simulink model "BLOCK_SEVEN_TAP_FILTER"  (R2022b)
settings: Solver=FixedStepDiscrete  StartTime=0.0  StopTime=10.0  RelTol=1e-3
libraries: dspsrcs4 x1
settings Model: DataTypeOverride=Off  Creator=saran  LastModifiedBy=saran
settings SolverCC: AlgebraicLoopSolver=TrustRegion
settings DataIOCC: LimitDataPoints=on  SaveOutput=off  SaveTime=off
settings OptimizationCC: BlockReduction=off  ConditionallyExecuteInputs=off  DefaultParameterBehavior=Inlined  DefaultUnderspecifiedDataType=single  LifeSpan=inf
settings DebuggingCC: AlgebraicLoopMsg=error  SingleTaskRateTransMsg=error  UnconnectedInputMsg=warning  UnconnectedOutputMsg=warning  UnconnectedLineMsg=warning  AllowSymbolicDim=off  StrictBusMsg=ErrorOnBusTreatedAsVector  SFUnexpectedBacktrackingDiag=warning  SFNoUnconditionalDefaultTransitionDiag=warning  SFExecutionAtInitializationDiag=none  SFMachineParentedDataDiag=warning  ArithmeticOperatorsInVariantConditions=warning
settings HardwareCC: ProdBitPerPointer=32  ProdBitPerSizeT=32  ProdBitPerPtrDiffT=32  ProdLargestAtomicFloat=None  ProdIntDivRoundTo=Undefined  ProdEndianess=Unspecified  ProdWordSize=32  ProdHWDeviceType=ASIC/FPGA->ASIC/FPGA  ProdEqTarget=off
settings ModelReferenceCC: EnableRefExpFcnMdlSchedulingChecks=on
settings SFSimCC: SimUseLocalCustomCode=off  CustomCodeUndefinedFunction=UseInterfaceOnly
settings RTWCC: RTWUseLocalCustomCode=off
settings CodeAppCC: StateflowObjectComments=on
settings GRTTargetCC: TargetLangStandard=C89/C90 (ANSI)
settings ConfigComp: CovScope=ReferencedModels  CovMetricSettings=dw  CovSaveCumulativeToWorkspaceVar=on  CovSaveSingleToWorkspaceVar=on  CovExternalEMLEnable=off  CovSFcnEnable=off

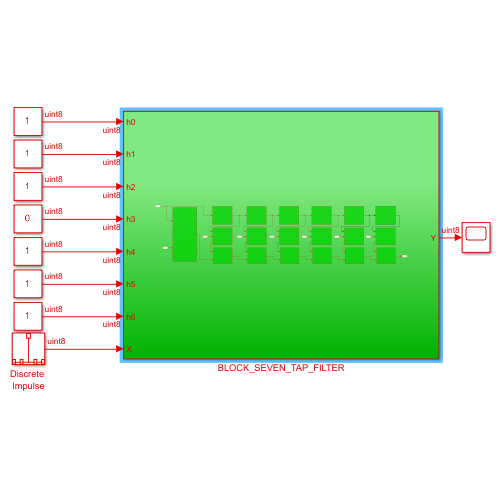
[thumbnail: Simulink's stored preview of the top-level diagram]
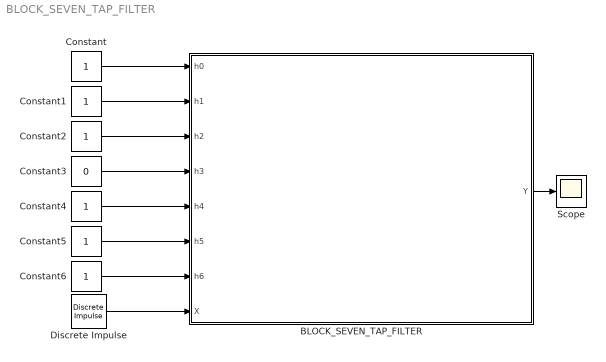
== system BLOCK_SEVEN_TAP_FILTER ==
  BLOCK_SEVEN_TAP_FILTER : Subsystem
  Constant{,1..2,4..6} (6 alike) : Constant  OutDataTypeStr=uint8  SampleTime=1
  Constant3 : Constant  Value=0  OutDataTypeStr=uint8  SampleTime=1
  Discrete Impulse : dspsrcs4/Discrete  Impulse  Delay=0  SampleTime=1  FrameSample=1  OutputFrames=off  dataType=uint8  isSigned=on  wordLen=16  udDataType=sfix(16)  fracBitsMode=Best precision  numFracBits=15  OutDataTypeStr=uint8  LastOutDataTypeStr=uint8
  Scope : Scope
  wires:
  Constant6/1 -> BLOCK_SEVEN_TAP_FILTER/7(h6)
  Constant/1 -> BLOCK_SEVEN_TAP_FILTER/1(h0)
  Constant1/1 -> BLOCK_SEVEN_TAP_FILTER/2(h1)
  Constant2/1 -> BLOCK_SEVEN_TAP_FILTER/3(h2)
  Constant3/1 -> BLOCK_SEVEN_TAP_FILTER/4(h3)
  Constant4/1 -> BLOCK_SEVEN_TAP_FILTER/5(h4)
  Constant5/1 -> BLOCK_SEVEN_TAP_FILTER/6(h5)
  Discrete Impulse/1 -> BLOCK_SEVEN_TAP_FILTER/8(X)
  BLOCK_SEVEN_TAP_FILTER/1(Y) -> Scope/1

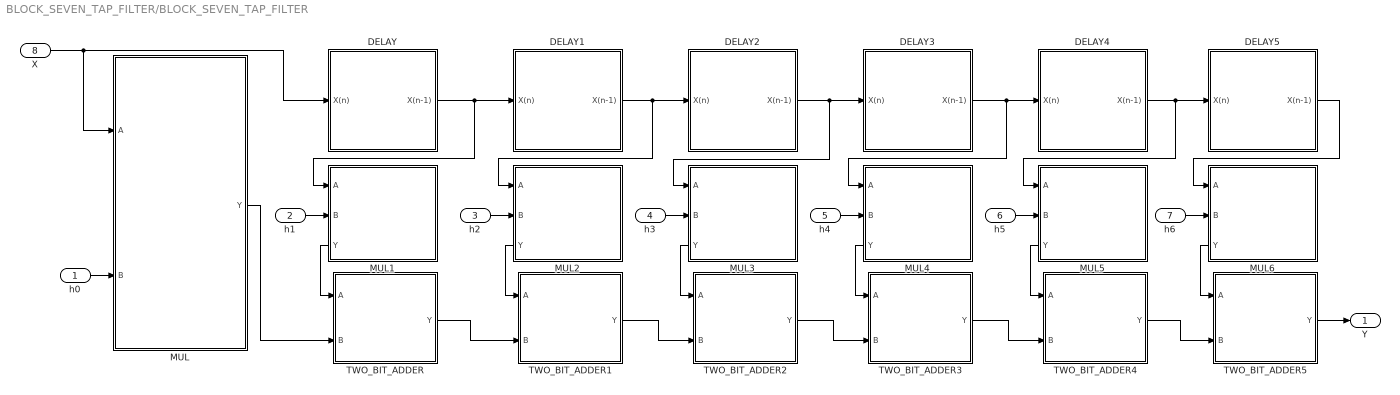
== system BLOCK_SEVEN_TAP_FILTER/BLOCK_SEVEN_TAP_FILTER ==
  h0 : Inport  OutDataTypeStr=uint8  SampleTime=1
  h1 : Inport  Port=2  OutDataTypeStr=uint8  SampleTime=1
  h2 : Inport  Port=3  OutDataTypeStr=uint8  SampleTime=1
  h3 : Inport  Port=4  OutDataTypeStr=uint8  SampleTime=1
  h4 : Inport  Port=5  OutDataTypeStr=uint8  SampleTime=1
  h5 : Inport  Port=6  OutDataTypeStr=uint8  SampleTime=1
  h6 : Inport  Port=7  OutDataTypeStr=uint8  SampleTime=1
  X : Inport  Port=8
  DELAY : Subsystem
  DELAY1 : Subsystem
  DELAY2 : Subsystem
  DELAY3 : Subsystem
  DELAY4 : Subsystem
  DELAY5 : Subsystem
  MUL : Subsystem
  MUL1 : Subsystem
      settings: PortSchema="{\"entries\":[{\"content\":{\"sides\":[{\"content\":{\"connectorIds\":[\"In1\",\"In2\",\"Out1\"]},\"type\":\"ConnectorPlacement.EquallySpacedRectSide\",\"uuid\":\"6d4885f8-73c5-433a-aace-af648e409d6b\"},{\"content\":{\"connectorIds\":[],\"side\":\"RIGHT\"},\"type\":\"ConnectorPlacement.EquallySpacedRectSide\",\"uuid\":\"836fe19b-05d9-46e4-8d72-fd0891ed8906\"},{\"content\":{\"connectorIds\":[],\"side\":\"TOP\"},\"type\":\"ConnectorPlacement.EquallySpacedRectSide\",\"uuid\":\"c1eb711e-365c-41f2-92fe-7283fb1d6e9c\"}]},\"type\":\"ConnectorPlacement.EquallySpacedConnector\",\"uuid\":\"b7c1d480-b729-42dd-8c7b-e0a62792d202\"}],\"packageUris\":[\"http://schema.mathworks.com/mf0/Connector/R2020b\"],\"version\":\"1.0\"}"
  MUL2 : Subsystem
      settings: PortSchema="{\"entries\":[{\"content\":{\"sides\":[{\"content\":{\"connectorIds\":[\"In1\",\"In2\",\"Out1\"]},\"type\":\"ConnectorPlacement.EquallySpacedRectSide\",\"uuid\":\"6d4885f8-73c5-433a-aace-af648e409d6b\"},{\"content\":{\"connectorIds\":[],\"side\":\"RIGHT\"},\"type\":\"ConnectorPlacement.EquallySpacedRectSide\",\"uuid\":\"836fe19b-05d9-46e4-8d72-fd0891ed8906\"},{\"content\":{\"connectorIds\":[],\"side\":\"TOP\"},\"type\":\"ConnectorPlacement.EquallySpacedRectSide\",\"uuid\":\"c1eb711e-365c-41f2-92fe-7283fb1d6e9c\"}]},\"type\":\"ConnectorPlacement.EquallySpacedConnector\",\"uuid\":\"b7c1d480-b729-42dd-8c7b-e0a62792d202\"}],\"packageUris\":[\"http://schema.mathworks.com/mf0/Connector/R2020b\"],\"version\":\"1.0\"}"
  MUL3 : Subsystem
      settings: PortSchema="{\"entries\":[{\"content\":{\"sides\":[{\"content\":{\"connectorIds\":[\"In1\",\"In2\",\"Out1\"]},\"type\":\"ConnectorPlacement.EquallySpacedRectSide\",\"uuid\":\"6d4885f8-73c5-433a-aace-af648e409d6b\"},{\"content\":{\"connectorIds\":[],\"side\":\"RIGHT\"},\"type\":\"ConnectorPlacement.EquallySpacedRectSide\",\"uuid\":\"836fe19b-05d9-46e4-8d72-fd0891ed8906\"},{\"content\":{\"connectorIds\":[],\"side\":\"TOP\"},\"type\":\"ConnectorPlacement.EquallySpacedRectSide\",\"uuid\":\"c1eb711e-365c-41f2-92fe-7283fb1d6e9c\"}]},\"type\":\"ConnectorPlacement.EquallySpacedConnector\",\"uuid\":\"b7c1d480-b729-42dd-8c7b-e0a62792d202\"}],\"packageUris\":[\"http://schema.mathworks.com/mf0/Connector/R2020b\"],\"version\":\"1.0\"}"
  MUL4 : Subsystem
      settings: PortSchema="{\"entries\":[{\"content\":{\"sides\":[{\"content\":{\"connectorIds\":[\"In1\",\"In2\",\"Out1\"]},\"type\":\"ConnectorPlacement.EquallySpacedRectSide\",\"uuid\":\"6d4885f8-73c5-433a-aace-af648e409d6b\"},{\"content\":{\"connectorIds\":[],\"side\":\"RIGHT\"},\"type\":\"ConnectorPlacement.EquallySpacedRectSide\",\"uuid\":\"836fe19b-05d9-46e4-8d72-fd0891ed8906\"},{\"content\":{\"connectorIds\":[],\"side\":\"TOP\"},\"type\":\"ConnectorPlacement.EquallySpacedRectSide\",\"uuid\":\"c1eb711e-365c-41f2-92fe-7283fb1d6e9c\"}]},\"type\":\"ConnectorPlacement.EquallySpacedConnector\",\"uuid\":\"b7c1d480-b729-42dd-8c7b-e0a62792d202\"}],\"packageUris\":[\"http://schema.mathworks.com/mf0/Connector/R2020b\"],\"version\":\"1.0\"}"
  MUL5 : Subsystem
      settings: PortSchema="{\"entries\":[{\"content\":{\"sides\":[{\"content\":{\"connectorIds\":[\"In1\",\"In2\",\"Out1\"]},\"type\":\"ConnectorPlacement.EquallySpacedRectSide\",\"uuid\":\"6d4885f8-73c5-433a-aace-af648e409d6b\"},{\"content\":{\"connectorIds\":[],\"side\":\"RIGHT\"},\"type\":\"ConnectorPlacement.EquallySpacedRectSide\",\"uuid\":\"836fe19b-05d9-46e4-8d72-fd0891ed8906\"},{\"content\":{\"connectorIds\":[],\"side\":\"TOP\"},\"type\":\"ConnectorPlacement.EquallySpacedRectSide\",\"uuid\":\"c1eb711e-365c-41f2-92fe-7283fb1d6e9c\"}]},\"type\":\"ConnectorPlacement.EquallySpacedConnector\",\"uuid\":\"b7c1d480-b729-42dd-8c7b-e0a62792d202\"}],\"packageUris\":[\"http://schema.mathworks.com/mf0/Connector/R2020b\"],\"version\":\"1.0\"}"
  MUL6 : Subsystem
      settings: PortSchema="{\"entries\":[{\"content\":{\"sides\":[{\"content\":{\"connectorIds\":[\"In1\",\"In2\",\"Out1\"]},\"type\":\"ConnectorPlacement.EquallySpacedRectSide\",\"uuid\":\"6d4885f8-73c5-433a-aace-af648e409d6b\"},{\"content\":{\"connectorIds\":[],\"side\":\"RIGHT\"},\"type\":\"ConnectorPlacement.EquallySpacedRectSide\",\"uuid\":\"836fe19b-05d9-46e4-8d72-fd0891ed8906\"},{\"content\":{\"connectorIds\":[],\"side\":\"TOP\"},\"type\":\"ConnectorPlacement.EquallySpacedRectSide\",\"uuid\":\"c1eb711e-365c-41f2-92fe-7283fb1d6e9c\"}]},\"type\":\"ConnectorPlacement.EquallySpacedConnector\",\"uuid\":\"b7c1d480-b729-42dd-8c7b-e0a62792d202\"}],\"packageUris\":[\"http://schema.mathworks.com/mf0/Connector/R2020b\"],\"version\":\"1.0\"}"
  TWO_BIT_ADDER : Subsystem
  TWO_BIT_ADDER1 : Subsystem
  TWO_BIT_ADDER2 : Subsystem
  TWO_BIT_ADDER3 : Subsystem
  TWO_BIT_ADDER4 : Subsystem
  TWO_BIT_ADDER5 : Subsystem
  Y : Outport  VectorParamsAs1DForOutWhenUnconnected=off
  wires:
  h1/1 -> MUL1/2(B)
  MUL1/1(Y) -> TWO_BIT_ADDER/1(A)
  MUL2/1(Y) -> TWO_BIT_ADDER1/1(A)
  h2/1 -> MUL2/2(B)
  MUL3/1(Y) -> TWO_BIT_ADDER2/1(A)
  h3/1 -> MUL3/2(B)
  MUL4/1(Y) -> TWO_BIT_ADDER3/1(A)
  h4/1 -> MUL4/2(B)
  MUL5/1(Y) -> TWO_BIT_ADDER4/1(A)
  h5/1 -> MUL5/2(B)
  MUL6/1(Y) -> TWO_BIT_ADDER5/1(A)
  h6/1 -> MUL6/2(B)
  MUL/1(Y) -> TWO_BIT_ADDER/2(B)
  DELAY/1(X(n-1)) -> MUL1/1(A), DELAY1/1(X(n))
  TWO_BIT_ADDER/1(Y) -> TWO_BIT_ADDER1/2(B)
  DELAY1/1(X(n-1)) -> DELAY2/1(X(n)), MUL2/1(A)
  DELAY2/1(X(n-1)) -> MUL3/1(A), DELAY3/1(X(n))
  DELAY3/1(X(n-1)) -> MUL4/1(A), DELAY4/1(X(n))
  TWO_BIT_ADDER1/1(Y) -> TWO_BIT_ADDER2/2(B)
  TWO_BIT_ADDER2/1(Y) -> TWO_BIT_ADDER3/2(B)
  TWO_BIT_ADDER3/1(Y) -> TWO_BIT_ADDER4/2(B)
  TWO_BIT_ADDER4/1(Y) -> TWO_BIT_ADDER5/2(B)
  X/1 -> DELAY/1(X(n)), MUL/1(A)
  h0/1 -> MUL/2(B)
  TWO_BIT_ADDER5/1(Y) -> Y/1
  DELAY4/1(X(n-1)) -> MUL5/1(A), DELAY5/1(X(n))
  DELAY5/1(X(n-1)) -> MUL6/1(A)

== system BLOCK_SEVEN_TAP_FILTER/BLOCK_SEVEN_TAP_FILTER/DELAY ==
  X(n) : Inport  OutDataTypeStr=uint8  SampleTime=1  LockScale=on
  Delay : Delay  DelayLength=1  InitialCondition=0
  X(n-1) : Outport  OutDataTypeStr=uint8  SampleTime=1  VectorParamsAs1DForOutWhenUnconnected=off  LockScale=on
  wires:
  X(n)/1 -> Delay/1
  Delay/1 -> X(n-1)/1

== system BLOCK_SEVEN_TAP_FILTER/BLOCK_SEVEN_TAP_FILTER/DELAY1 ==
  X(n) : Inport  OutDataTypeStr=uint8  SampleTime=1  LockScale=on
  Delay : Delay  DelayLength=1  InitialCondition=0
  X(n-1) : Outport  OutDataTypeStr=uint8  SampleTime=1  VectorParamsAs1DForOutWhenUnconnected=off  LockScale=on
  wires:
  X(n)/1 -> Delay/1
  Delay/1 -> X(n-1)/1

== system BLOCK_SEVEN_TAP_FILTER/BLOCK_SEVEN_TAP_FILTER/DELAY2 ==
  X(n) : Inport  OutDataTypeStr=uint8  SampleTime=1  LockScale=on
  Delay : Delay  DelayLength=1  InitialCondition=0
  X(n-1) : Outport  OutDataTypeStr=uint8  SampleTime=1  VectorParamsAs1DForOutWhenUnconnected=off  LockScale=on
  wires:
  X(n)/1 -> Delay/1
  Delay/1 -> X(n-1)/1

== system BLOCK_SEVEN_TAP_FILTER/BLOCK_SEVEN_TAP_FILTER/DELAY3 ==
  X(n) : Inport  OutDataTypeStr=uint8  SampleTime=1  LockScale=on
  Delay : Delay  DelayLength=1  InitialCondition=0
  X(n-1) : Outport  OutDataTypeStr=uint8  SampleTime=1  VectorParamsAs1DForOutWhenUnconnected=off  LockScale=on
  wires:
  X(n)/1 -> Delay/1
  Delay/1 -> X(n-1)/1

== system BLOCK_SEVEN_TAP_FILTER/BLOCK_SEVEN_TAP_FILTER/DELAY4 ==
  X(n) : Inport  OutDataTypeStr=uint8  SampleTime=1  LockScale=on
  Delay : Delay  DelayLength=1  InitialCondition=0
  X(n-1) : Outport  OutDataTypeStr=uint8  SampleTime=1  VectorParamsAs1DForOutWhenUnconnected=off  LockScale=on
  wires:
  X(n)/1 -> Delay/1
  Delay/1 -> X(n-1)/1

== system BLOCK_SEVEN_TAP_FILTER/BLOCK_SEVEN_TAP_FILTER/DELAY5 ==
  X(n) : Inport  OutDataTypeStr=uint8  SampleTime=1  LockScale=on
  Delay : Delay  DelayLength=1  InitialCondition=0
  X(n-1) : Outport  OutDataTypeStr=uint8  SampleTime=1  VectorParamsAs1DForOutWhenUnconnected=off  LockScale=on
  wires:
  X(n)/1 -> Delay/1
  Delay/1 -> X(n-1)/1

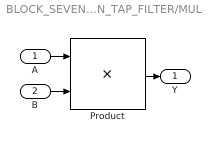
== system BLOCK_SEVEN_TAP_FILTER/BLOCK_SEVEN_TAP_FILTER/MUL ==
  A : Inport  OutDataTypeStr=uint8  SampleTime=1
  B : Inport  Port=2  OutDataTypeStr=uint8  SampleTime=1
  Product : Product  OutDataTypeStr=uint8  LockScale=on
  Y : Outport  OutDataTypeStr=uint8  SampleTime=1  VectorParamsAs1DForOutWhenUnconnected=off
  wires:
  A/1 -> Product/1
  Product/1 -> Y/1
  B/1 -> Product/2

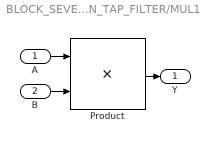
== system BLOCK_SEVEN_TAP_FILTER/BLOCK_SEVEN_TAP_FILTER/MUL1 ==
  A : Inport  OutDataTypeStr=uint8  SampleTime=1
  B : Inport  Port=2  OutDataTypeStr=uint8  SampleTime=1
  Product : Product  OutDataTypeStr=uint8  LockScale=on
  Y : Outport  OutDataTypeStr=uint8  SampleTime=1  VectorParamsAs1DForOutWhenUnconnected=off
  wires:
  A/1 -> Product/1
  Product/1 -> Y/1
  B/1 -> Product/2

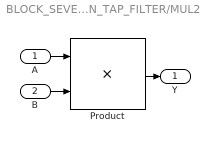
== system BLOCK_SEVEN_TAP_FILTER/BLOCK_SEVEN_TAP_FILTER/MUL2 ==
  A : Inport  OutDataTypeStr=uint8  SampleTime=1
  B : Inport  Port=2  OutDataTypeStr=uint8  SampleTime=1
  Product : Product  OutDataTypeStr=uint8  LockScale=on
  Y : Outport  OutDataTypeStr=uint8  SampleTime=1  VectorParamsAs1DForOutWhenUnconnected=off
  wires:
  A/1 -> Product/1
  Product/1 -> Y/1
  B/1 -> Product/2

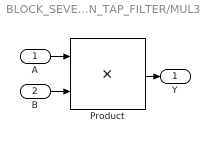
== system BLOCK_SEVEN_TAP_FILTER/BLOCK_SEVEN_TAP_FILTER/MUL3 ==
  A : Inport  OutDataTypeStr=uint8  SampleTime=1
  B : Inport  Port=2  OutDataTypeStr=uint8  SampleTime=1
  Product : Product  OutDataTypeStr=uint8  LockScale=on
  Y : Outport  OutDataTypeStr=uint8  SampleTime=1  VectorParamsAs1DForOutWhenUnconnected=off
  wires:
  A/1 -> Product/1
  Product/1 -> Y/1
  B/1 -> Product/2

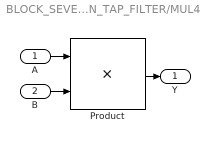
== system BLOCK_SEVEN_TAP_FILTER/BLOCK_SEVEN_TAP_FILTER/MUL4 ==
  A : Inport  OutDataTypeStr=uint8  SampleTime=1
  B : Inport  Port=2  OutDataTypeStr=uint8  SampleTime=1
  Product : Product  OutDataTypeStr=uint8  LockScale=on
  Y : Outport  OutDataTypeStr=uint8  SampleTime=1  VectorParamsAs1DForOutWhenUnconnected=off
  wires:
  A/1 -> Product/1
  Product/1 -> Y/1
  B/1 -> Product/2

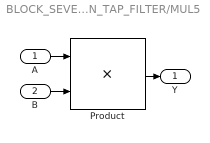
== system BLOCK_SEVEN_TAP_FILTER/BLOCK_SEVEN_TAP_FILTER/MUL5 ==
  A : Inport  OutDataTypeStr=uint8  SampleTime=1
  B : Inport  Port=2  OutDataTypeStr=uint8  SampleTime=1
  Product : Product  OutDataTypeStr=uint8  LockScale=on
  Y : Outport  OutDataTypeStr=uint8  SampleTime=1  VectorParamsAs1DForOutWhenUnconnected=off
  wires:
  A/1 -> Product/1
  Product/1 -> Y/1
  B/1 -> Product/2

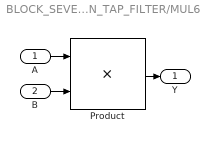
== system BLOCK_SEVEN_TAP_FILTER/BLOCK_SEVEN_TAP_FILTER/MUL6 ==
  A : Inport  OutDataTypeStr=uint8  SampleTime=1
  B : Inport  Port=2  OutDataTypeStr=uint8  SampleTime=1
  Product : Product  OutDataTypeStr=uint8  LockScale=on
  Y : Outport  OutDataTypeStr=uint8  SampleTime=1  VectorParamsAs1DForOutWhenUnconnected=off
  wires:
  A/1 -> Product/1
  Product/1 -> Y/1
  B/1 -> Product/2

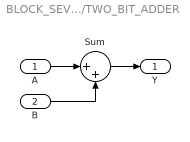
== system BLOCK_SEVEN_TAP_FILTER/BLOCK_SEVEN_TAP_FILTER/TWO_BIT_ADDER ==
  A : Inport  OutDataTypeStr=uint8
  B : Inport  Port=2  OutDataTypeStr=uint8  SampleTime=1
  Sum : Sum  Inputs=|++  OutDataTypeStr=uint8  LockScale=on
  Y : Outport  OutDataTypeStr=uint8  SampleTime=1  VectorParamsAs1DForOutWhenUnconnected=off
  wires:
  Sum/1 -> Y/1
  A/1 -> Sum/1
  B/1 -> Sum/2

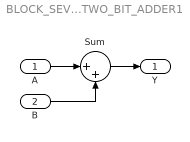
== system BLOCK_SEVEN_TAP_FILTER/BLOCK_SEVEN_TAP_FILTER/TWO_BIT_ADDER1 ==
  A : Inport  OutDataTypeStr=uint8
  B : Inport  Port=2  OutDataTypeStr=uint8  SampleTime=1
  Sum : Sum  Inputs=|++  OutDataTypeStr=uint8  LockScale=on
  Y : Outport  OutDataTypeStr=uint8  SampleTime=1  VectorParamsAs1DForOutWhenUnconnected=off
  wires:
  Sum/1 -> Y/1
  A/1 -> Sum/1
  B/1 -> Sum/2

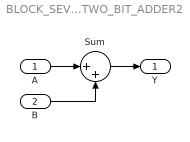
== system BLOCK_SEVEN_TAP_FILTER/BLOCK_SEVEN_TAP_FILTER/TWO_BIT_ADDER2 ==
  A : Inport  OutDataTypeStr=uint8
  B : Inport  Port=2  OutDataTypeStr=uint8  SampleTime=1
  Sum : Sum  Inputs=|++  OutDataTypeStr=uint8  LockScale=on
  Y : Outport  OutDataTypeStr=uint8  SampleTime=1  VectorParamsAs1DForOutWhenUnconnected=off
  wires:
  Sum/1 -> Y/1
  A/1 -> Sum/1
  B/1 -> Sum/2

== system BLOCK_SEVEN_TAP_FILTER/BLOCK_SEVEN_TAP_FILTER/TWO_BIT_ADDER3 ==
  A : Inport  OutDataTypeStr=uint8
  B : Inport  Port=2  OutDataTypeStr=uint8  SampleTime=1
  Sum : Sum  Inputs=|++  OutDataTypeStr=uint8  LockScale=on
  Y : Outport  OutDataTypeStr=uint8  SampleTime=1  VectorParamsAs1DForOutWhenUnconnected=off
  wires:
  Sum/1 -> Y/1
  A/1 -> Sum/1
  B/1 -> Sum/2

== system BLOCK_SEVEN_TAP_FILTER/BLOCK_SEVEN_TAP_FILTER/TWO_BIT_ADDER4 ==
  A : Inport  OutDataTypeStr=uint8
  B : Inport  Port=2  OutDataTypeStr=uint8  SampleTime=1
  Sum : Sum  Inputs=|++  OutDataTypeStr=uint8  LockScale=on
  Y : Outport  OutDataTypeStr=uint8  SampleTime=1  VectorParamsAs1DForOutWhenUnconnected=off
  wires:
  Sum/1 -> Y/1
  A/1 -> Sum/1
  B/1 -> Sum/2

== system BLOCK_SEVEN_TAP_FILTER/BLOCK_SEVEN_TAP_FILTER/TWO_BIT_ADDER5 ==
  A : Inport  OutDataTypeStr=uint8
  B : Inport  Port=2  OutDataTypeStr=uint8  SampleTime=1
  Sum : Sum  Inputs=|++  OutDataTypeStr=uint8  LockScale=on
  Y : Outport  OutDataTypeStr=uint8  SampleTime=1  VectorParamsAs1DForOutWhenUnconnected=off
  wires:
  Sum/1 -> Y/1
  A/1 -> Sum/1
  B/1 -> Sum/2
